simulink model "inverted_pendulum_"  (R2024b)
settings: Solver=VariableStepAuto  StartTime=0.0  StopTime=100  RelTol=1e-3
values from neighbouring files (symbols this model uses):
  g = 9.8    [inverted_script.m]    (also in tanks_variable.m = 9.82)
  K = acker(A,B,nv_poles)    [inverted_script.m]
  l = 0.5    [inverted_script.m]
  M = 2    [inverted_script.m]
  m = 0.5    [inverted_script.m]
settings Model: Creator=thomas  LastModifiedBy=thomas

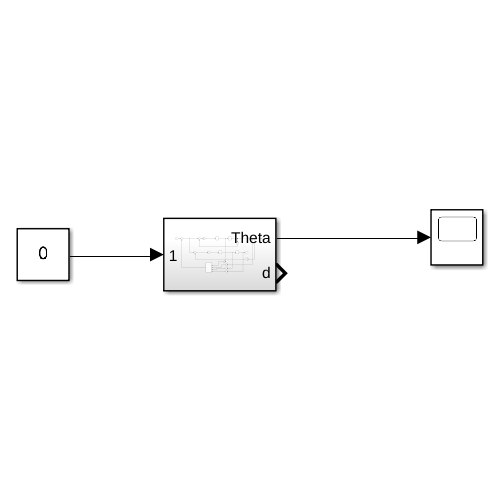
[thumbnail: Simulink's stored preview of the top-level diagram]
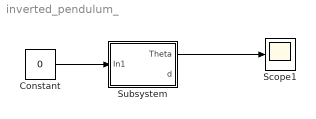
== system inverted_pendulum_ ==
  Constant : Constant  Value=0
  Scope1 : Scope
  Subsystem : Subsystem
  wires:
  Subsystem/1(Theta) -> Scope1/1
  Constant/1 -> Subsystem/1(In1)

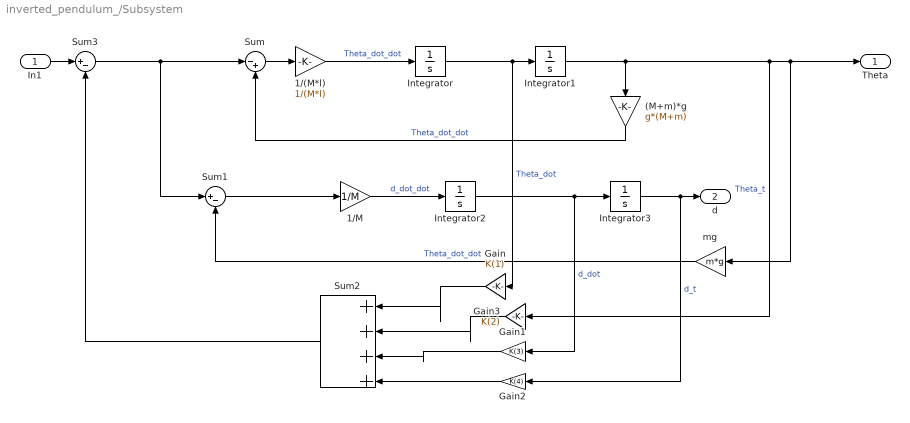
== system inverted_pendulum_/Subsystem ==
  In1 : Inport
  (M+m)*g : Gain  Gain=g*(M+m)
  1/(M*l) : Gain  Gain=1/(M*l)
  1/M : Gain  Gain=1/M
  Gain : Gain  Gain=K(1)
  Gain1 : Gain  Gain=K(3)
  Gain2 : Gain  Gain=K(4)
  Gain3 : Gain  Gain=K(2)
  Integrator : Integrator
  Integrator1 : Integrator  InitialCondition=0.7
  Integrator2 : Integrator
  Integrator3 : Integrator
  Sum : Sum  Inputs=|-+
  Sum1 : Sum  Inputs=|+-
  Sum2 : Sum  Inputs=|++++
  Sum3 : Sum  Inputs=|+-
  mg : Gain  Gain=m*g
  Theta : Outport
  d : Outport  Port=2
  wires:
  Integrator/1 -> Gain/1, Integrator1/1  "Theta_dot"
  Integrator2/1 -> Gain1/1, Integrator3/1  "d_dot"
  Sum1/1 -> 1/M/1
  Sum/1 -> 1/(M*l)/1
  1/(M*l)/1 -> Integrator/1  "Theta_dot_dot"
  1/M/1 -> Integrator2/1  "d_dot_dot"
  Integrator1/1 -> Gain3/1, Theta/1, mg/1, (M+m)*g/1  "Theta_t"
  Integrator3/1 -> Gain2/1, d/1  "d_t"
  (M+m)*g/1 -> Sum/2  "Theta_dot_dot"
  mg/1 -> Sum1/2  "Theta_dot_dot"
  Gain/1 -> Sum2/1
  Gain3/1 -> Sum2/2
  Gain1/1 -> Sum2/3
  Gain2/1 -> Sum2/4
  Sum2/1 -> Sum3/2
  In1/1 -> Sum3/1
  Sum3/1 -> Sum1/1, Sum/1
